simulink model "adcs_sim_finch"  (R2025b)
settings: Solver=VariableStepAuto  StartTime=0.0  StopTime=10.0  RelTol=1e-3
PreLoadFcn:
  | run("sim_config.m")
undefined symbols (not defined in the file or in its folder): MU_EARTH_KM3PS2, sc
libraries: simulink x11
settings Model: Creator=alex  LastModifiedBy=alex

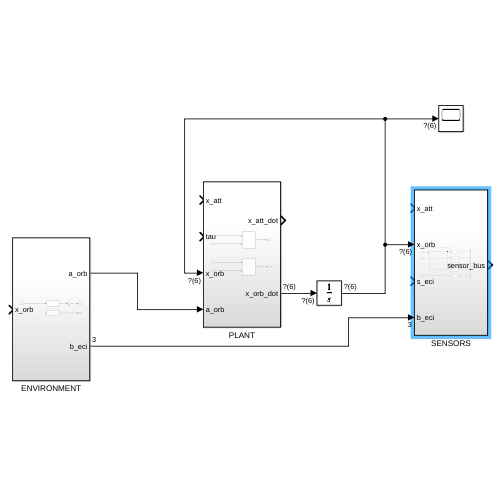
[thumbnail: Simulink's stored preview of the top-level diagram]
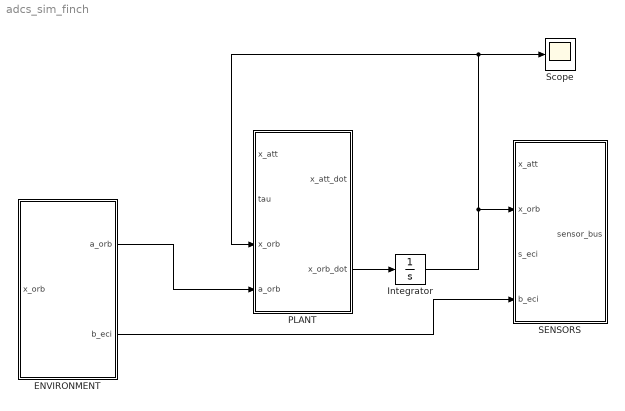
== system adcs_sim_finch ==
  ENVIRONMENT : Subsystem
  Integrator : Integrator
  PLANT : Subsystem
  SENSORS : Subsystem
  Scope : Scope
  wires:
  ENVIRONMENT/1(a_orb) -> PLANT/4(a_orb)
  PLANT/2(x_orb_dot) -> Integrator/1
  Integrator/1 -> SENSORS/2(x_orb), Scope/1, PLANT/3(x_orb)
  ENVIRONMENT/2(b_eci) -> SENSORS/4(b_eci)

== system adcs_sim_finch/ENVIRONMENT ==
  x_orb : Inport
  GEOMAGNETISM : Subsystem
  GRAVITY : Subsystem
  Sum : Sum  Inputs=|++
  a_orb : Outport
  b_eci : Outport  Port=2
  wires:
  x_orb/1 -> GRAVITY/1(x_orb)
  GRAVITY/1(a_grav) -> Sum/1
  Sum/1 -> a_orb/1
  GEOMAGNETISM/1(b) -> b_eci/1

== system adcs_sim_finch/PLANT ==
  x_att : Inport
  tau : Inport  Port=2
  x_orb : Inport  Port=3
  a_orb : Inport  Port=4
  ATTITUDE : Subsystem
  ORBIT : Subsystem
  x_att_dot : Outport
  x_orb_dot : Outport  Port=2
  wires:
  x_att/1 -> ATTITUDE/1(x)
  tau/1 -> ATTITUDE/2(tau)
  x_orb/1 -> ORBIT/1(x_orb)
  ATTITUDE/1(x_dot) -> x_att_dot/1
  ORBIT/1(x_orb_dot) -> x_orb_dot/1
  a_orb/1 -> ORBIT/2(a_orb)

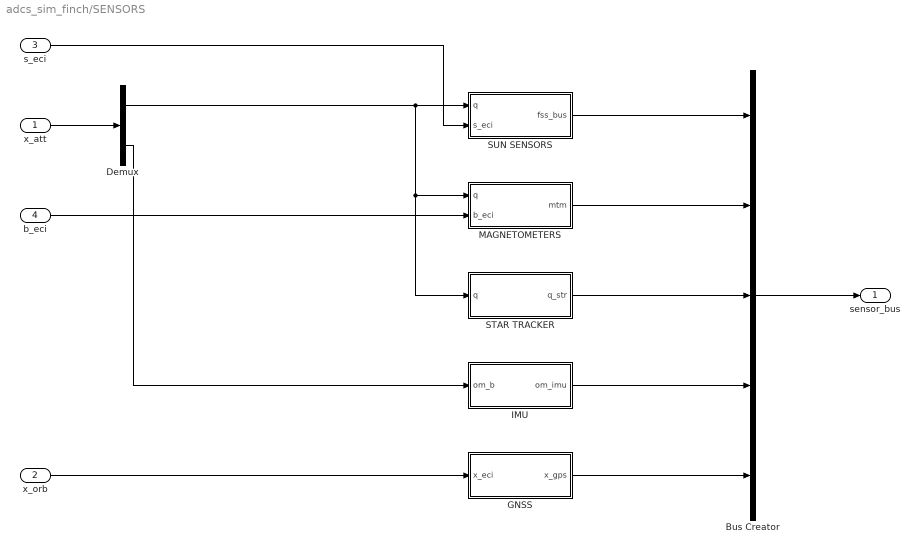
== system adcs_sim_finch/SENSORS ==
  x_att : Inport
  x_orb : Inport  Port=2
  s_eci : Inport  Port=3
  b_eci : Inport  Port=4
  Bus Creator : BusCreator  Inputs=5
  Demux : Demux  Outputs=[4, 3]
  GNSS : Subsystem
  IMU : Subsystem
  MAGNETOMETERS : Subsystem
  STAR TRACKER : Subsystem
  SUN SENSORS : Subsystem
  sensor_bus : Outport
  wires:
  x_att/1 -> Demux/1
  Demux/1 -> STAR TRACKER/1(q), MAGNETOMETERS/1(q), SUN SENSORS/1(q)
  Demux/2 -> IMU/1(om_b)
  x_orb/1 -> GNSS/1(x_eci)
  s_eci/1 -> SUN SENSORS/2(s_eci)
  b_eci/1 -> MAGNETOMETERS/2(b_eci)
  SUN SENSORS/1(fss_bus) -> Bus Creator/1
  GNSS/1(x_gps) -> Bus Creator/5
  IMU/1(om_imu) -> Bus Creator/4
  STAR TRACKER/1(q_str) -> Bus Creator/3
  MAGNETOMETERS/1(mtm) -> Bus Creator/2
  Bus Creator/1 -> sensor_bus/1

== system adcs_sim_finch/ENVIRONMENT/GEOMAGNETISM ==
  x_orb : Inport
  PLACEHOLDER : Constant  Value=[60; 0; 0]
  b : Outport
  wires:
  PLACEHOLDER/1 -> b/1

== system adcs_sim_finch/ENVIRONMENT/GRAVITY ==
  x_orb : Inport
  J2 : Subsystem
  Mux : Mux  Inputs=2
  a_grav : Outport
  wires:
  x_orb/1 -> J2/1(x_orb)
  J2/1(p) -> Mux/1
  Mux/1 -> a_grav/1

== system adcs_sim_finch/PLANT/ATTITUDE ==
  x : Inport
  tau : Inport  Port=2
  DYNAMICS : Subsystem
  Demux : Demux  Outputs=2
  KINEMATICS : Subsystem
  Mux : Mux  Inputs=2
  x_dot : Outport
  wires:
  x/1 -> Demux/1
  Demux/1 -> KINEMATICS/1(q)  "q"
  Demux/2 -> KINEMATICS/2(om_b), DYNAMICS/1(om_b)  "om_b"
  tau/1 -> DYNAMICS/2(tau)
  KINEMATICS/1(q_dot) -> Mux/1
  DYNAMICS/1(om_b_dot) -> Mux/2
  Mux/1 -> x_dot/1

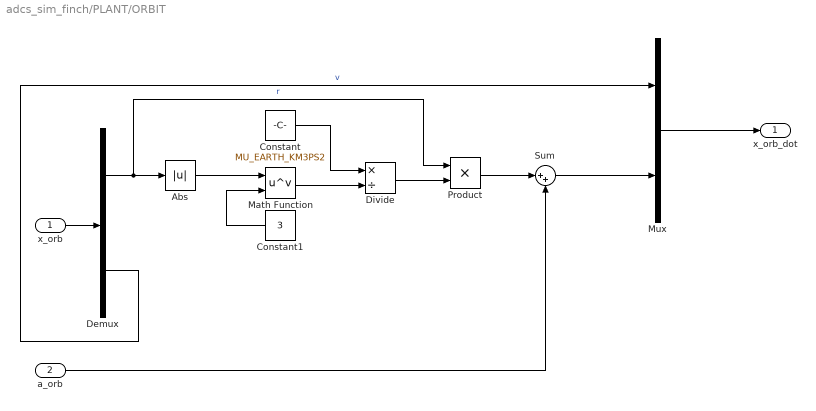
== system adcs_sim_finch/PLANT/ORBIT ==
  x_orb : Inport
  a_orb : Inport  Port=2
  Abs : Abs  SaturateOnIntegerOverflow=off
  Constant : Constant  Value=MU_EARTH_KM3PS2
  Constant1 : Constant  Value=3
  Demux : Demux  Outputs=[3, 3]
  Divide : Product  Inputs=*/
  Math Function : Math  Operator=pow
  Mux : Mux  Inputs=2
  Product : Product
  Sum : Sum  Inputs=|++
  x_orb_dot : Outport
  wires:
  x_orb/1 -> Demux/1
  Mux/1 -> x_orb_dot/1
  Constant1/1 -> Math Function/2
  Demux/1 -> Product/1, Abs/1  "r"
  Abs/1 -> Math Function/1
  Math Function/1 -> Divide/2
  Constant/1 -> Divide/1
  Divide/1 -> Product/2
  Product/1 -> Sum/1
  a_orb/1 -> Sum/2
  Sum/1 -> Mux/2
  Demux/2 -> Mux/1  "v"

== system adcs_sim_finch/SENSORS/GNSS ==
  x_eci : Inport
  Band-Limited White Noise : simulink/Sources/Band-Limited White Noise  Cov=sc.gps.obj.cov ./ (1 / sc.gps.obj.rate)  Ts=1 / sc.gps.obj.rate  seed=[23341]
  Sum : Sum  Inputs=|++
  x_gps : Outport
  wires:
  x_eci/1 -> Sum/1
  Sum/1 -> x_gps/1

== system adcs_sim_finch/SENSORS/IMU ==
  om_b : Inport
  Band-Limited White Noise : simulink/Sources/Band-Limited White Noise  Cov=sc.imu.obj.bias_instability.^2 ./ (1 ./ sc.imu.obj.rate)  Ts=1 / sc.imu.obj.rate  seed=[23341]
  Band-Limited White Noise1 : simulink/Sources/Band-Limited White Noise  Cov=sc.imu.obj.arw.^2  Ts=1 / sc.imu.obj.rate  seed=[23341]
  Integrator : Integrator
  Product : Product  Multiplication=Matrix(*)
  Sum : Sum  Inputs=+++
  sc.imu.dcm : Constant  Value=sc.imu.dcm
  om_imu : Outport
  wires:
  om_b/1 -> Product/2
  sc.imu.dcm/1 -> Product/1
  Product/1 -> Sum/2
  Integrator/1 -> Sum/3  "bias"
  Sum/1 -> om_imu/1

== system adcs_sim_finch/SENSORS/MAGNETOMETERS ==
  q : Inport
  b_eci : Inport  Port=2
  MTM1 : Subsystem
  mtm : Outport
  wires:
  q/1 -> MTM1/1(q)
  b_eci/1 -> MTM1/2(b_eci)
  MTM1/1(b_s) -> mtm/1

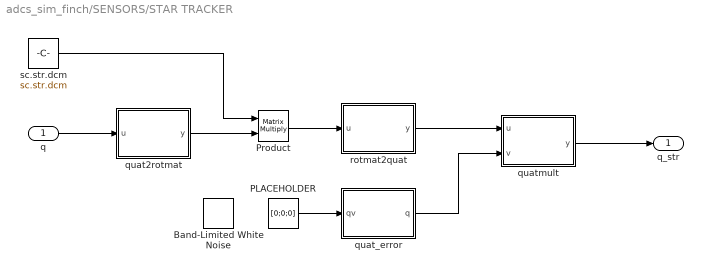
== system adcs_sim_finch/SENSORS/STAR TRACKER ==
  q : Inport
  Band-Limited White Noise : simulink/Sources/Band-Limited White Noise  Cov=sc.str.obj.cov  Ts=1 / sc.str.obj.rate  seed=[23341]
  PLACEHOLDER : Constant  Value=[0;0;0]
  Product : Product  Multiplication=Matrix(*)
  quat2rotmat : MATLAB Function  TreatAsAtomicUnit=on
  quat_error : MATLAB Function  TreatAsAtomicUnit=on
  quatmult : MATLAB Function  TreatAsAtomicUnit=on
  rotmat2quat : MATLAB Function  TreatAsAtomicUnit=on
  sc.str.dcm : Constant  Value=sc.str.dcm
  q_str : Outport
  wires:
  q/1 -> quat2rotmat/1(u)
  quat2rotmat/1(y) -> Product/2
  sc.str.dcm/1 -> Product/1
  Product/1 -> rotmat2quat/1(u)
  rotmat2quat/1(y) -> quatmult/1(u)
  quat_error/1(q) -> quatmult/2(v)
  quatmult/1(y) -> q_str/1
  PLACEHOLDER/1 -> quat_error/1(qv)

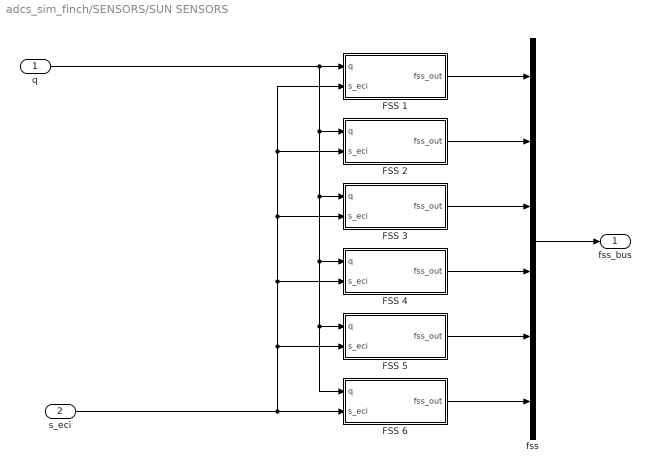
== system adcs_sim_finch/SENSORS/SUN SENSORS ==
  q : Inport
  s_eci : Inport  Port=2
  FSS 1 : Subsystem
  FSS 2 : Subsystem
  FSS 3 : Subsystem
  FSS 4 : Subsystem
  FSS 5 : Subsystem
  FSS 6 : Subsystem
  fss : BusCreator  Inputs=6
  fss_bus : Outport
  wires:
  FSS 1/1(fss_out) -> fss/1
  FSS 2/1(fss_out) -> fss/2
  FSS 3/1(fss_out) -> fss/3
  FSS 4/1(fss_out) -> fss/4
  FSS 5/1(fss_out) -> fss/5
  FSS 6/1(fss_out) -> fss/6
  q/1 -> FSS 5/1(q), FSS 6/1(q), FSS 4/1(q), FSS 3/1(q), FSS 2/1(q), FSS 1/1(q)
  s_eci/1 -> FSS 1/2(s_eci), FSS 2/2(s_eci), FSS 3/2(s_eci), FSS 4/2(s_eci), FSS 5/2(s_eci), FSS 6/2(s_eci)
  fss/1 -> fss_bus/1

== system adcs_sim_finch/ENVIRONMENT/GRAVITY/J2 ==
  x_orb : Inport
  J2 acceleration : MATLAB Function  TreatAsAtomicUnit=on
  p : Outport
  wires:
  x_orb/1 -> J2 acceleration/1(x)
  J2 acceleration/1(p) -> p/1

== system adcs_sim_finch/PLANT/ATTITUDE/DYNAMICS ==
  om_b : Inport
  tau : Inport  Port=2
  Constant : Constant  Value=sc.moi
  Product : Product  Inputs=3  Multiplication=Matrix(*)
  Product1 : Product  Multiplication=Matrix(*)
  Sum : Sum  Inputs=-+|
  sc.moi_inv : Constant  Value=sc.moi_inv
  skew3 : MATLAB Function  TreatAsAtomicUnit=on
  om_b_dot : Outport
  wires:
  om_b/1 -> Product/2, skew3/1(u)
  skew3/1(y) -> Product/3
  Constant/1 -> Product/1
  tau/1 -> Sum/2
  Product/1 -> Sum/1
  Sum/1 -> Product1/2
  sc.moi_inv/1 -> Product1/1
  Product1/1 -> om_b_dot/1

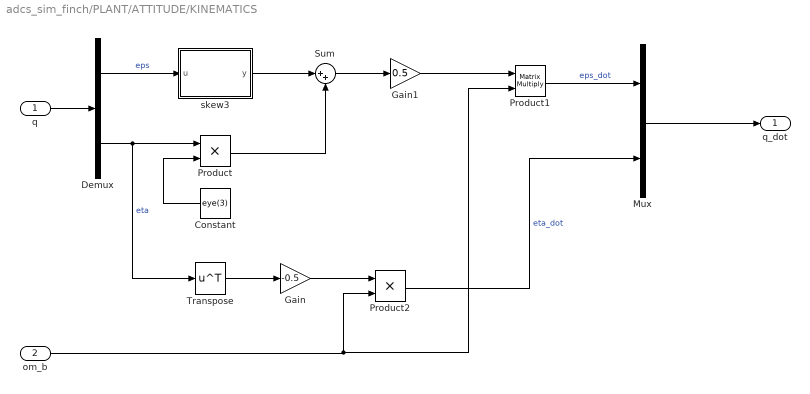
== system adcs_sim_finch/PLANT/ATTITUDE/KINEMATICS ==
  q : Inport
  om_b : Inport  Port=2
  Constant : Constant  Value=eye(3)
  Demux : Demux  Outputs=[3, 1]
  Gain : Gain  Gain=-0.5
  Gain1 : Gain  Gain=0.5
  Mux : Mux  Inputs=2
  Product : Product
  Product1 : Product  Multiplication=Matrix(*)
  Product2 : Product
  Sum : Sum  Inputs=|++
  Transpose : Math  Operator=transpose
  skew3 : MATLAB Function  TreatAsAtomicUnit=on
  q_dot : Outport
  wires:
  q/1 -> Demux/1
  Transpose/1 -> Gain/1
  Demux/1 -> skew3/1(u)  "eps"
  skew3/1(y) -> Sum/1
  Demux/2 -> Transpose/1, Product/1  "eta"
  Constant/1 -> Product/2
  Product/1 -> Sum/2
  Sum/1 -> Gain1/1
  Gain1/1 -> Product1/1
  Product1/1 -> Mux/1  "eps_dot"
  Gain/1 -> Product2/1
  om_b/1 -> Product1/2, Product2/2
  Product2/1 -> Mux/2  "eta_dot"
  Mux/1 -> q_dot/1

== system adcs_sim_finch/SENSORS/MAGNETOMETERS/MTM1 ==
  q : Inport
  b_eci : Inport  Port=2
  Band-Limited White Noise : simulink/Sources/Band-Limited White Noise  Cov=sc.mtm1.obj.cov ./ (1 / sc.mtm1.obj.rate)  Ts=1 / sc.mtm1.obj.rate  seed=[23341]
  Product : Product  Multiplication=Matrix(*)
  Product1 : Product  Multiplication=Matrix(*)
  Saturation : Saturate  UpperLimit=sc.mtm1.obj.range(2)  LowerLimit=sc.mtm1.obj.range(1)
  Sum : Sum  Inputs=|++
  quat2rotmat : MATLAB Function  TreatAsAtomicUnit=on
  sc.mtm1.dcm : Constant  Value=sc.mtm1.dcm
  b_s : Outport
  wires:
  q/1 -> quat2rotmat/1(u)
  Product/1 -> Product1/2
  sc.mtm1.dcm/1 -> Product1/1
  Product1/1 -> Sum/1
  Sum/1 -> Saturation/1
  Saturation/1 -> b_s/1
  b_eci/1 -> Product/2
  quat2rotmat/1(y) -> Product/1

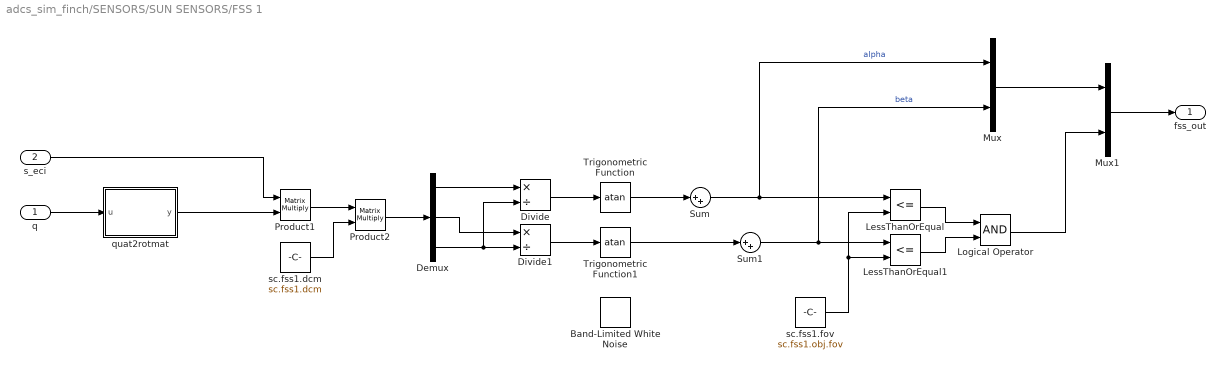
== system adcs_sim_finch/SENSORS/SUN SENSORS/FSS 1 ==
  q : Inport
  s_eci : Inport  Port=2
  Band-Limited White Noise : simulink/Sources/Band-Limited White Noise  Cov=sc.fss1.obj.cov ./ (1 / sc.fss1.obj.rate)  Ts=1 / sc.fss1.obj.rate  seed=[23341]
  Demux : Demux  Outputs=3
  Divide : Product  Inputs=*/
  Divide1 : Product  Inputs=*/
  LessThanOrEqual : RelationalOperator  Operator=<=  OutDataTypeStr=boolean  RndMeth=Simplest  InputSameDT=off
  LessThanOrEqual1 : RelationalOperator  Operator=<=  OutDataTypeStr=boolean  RndMeth=Simplest  InputSameDT=off
  Logical Operator : Logic  AllPortsSameDT=off  OutDataTypeStr=boolean
  Mux : Mux  Inputs=2
  Mux1 : Mux  Inputs=2
  Product1 : Product  Multiplication=Matrix(*)
  Product2 : Product  Multiplication=Matrix(*)
  Sum : Sum  Inputs=|++
  Sum1 : Sum  Inputs=|++
  Trigonometric Function : Trigonometry  Operator=atan
  Trigonometric Function1 : Trigonometry  Operator=atan
  quat2rotmat : MATLAB Function  TreatAsAtomicUnit=on
  sc.fss1.dcm : Constant  Value=sc.fss1.dcm
  sc.fss1.fov : Constant  Value=sc.fss1.obj.fov
  fss_out : Outport
  wires:
  q/1 -> quat2rotmat/1(u)
  quat2rotmat/1(y) -> Product1/2
  sc.fss1.dcm/1 -> Product2/2
  s_eci/1 -> Product1/1
  Product1/1 -> Product2/1
  Product2/1 -> Demux/1
  Demux/1 -> Divide/1
  Demux/3 -> Divide1/2, Divide/2
  Divide/1 -> Trigonometric Function/1
  Demux/2 -> Divide1/1
  Divide1/1 -> Trigonometric Function1/1
  Trigonometric Function/1 -> Sum/1
  Trigonometric Function1/1 -> Sum1/1
  Sum/1 -> Mux/1, LessThanOrEqual/1  "alpha"
  sc.fss1.fov/1 -> LessThanOrEqual1/2, LessThanOrEqual/2
  Sum1/1 -> Mux/2, LessThanOrEqual1/1  "beta"
  LessThanOrEqual/1 -> Logical Operator/1
  LessThanOrEqual1/1 -> Logical Operator/2
  Mux/1 -> Mux1/1
  Logical Operator/1 -> Mux1/2
  Mux1/1 -> fss_out/1

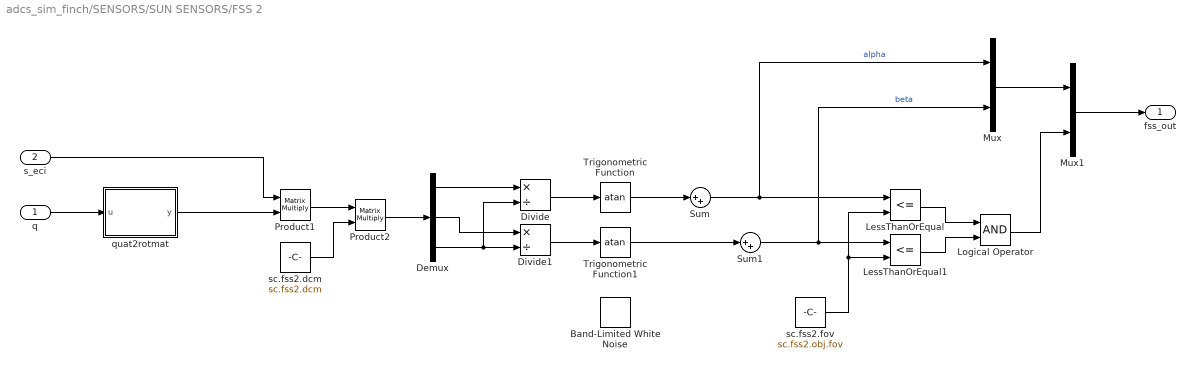
== system adcs_sim_finch/SENSORS/SUN SENSORS/FSS 2 ==
  q : Inport
  s_eci : Inport  Port=2
  Band-Limited White Noise : simulink/Sources/Band-Limited White Noise  Cov=sc.fss2.obj.cov ./ (1 / sc.fss2.obj.rate)  Ts=1 / sc.fss2.obj.rate  seed=[23341]
  Demux : Demux  Outputs=3
  Divide : Product  Inputs=*/
  Divide1 : Product  Inputs=*/
  LessThanOrEqual : RelationalOperator  Operator=<=  OutDataTypeStr=boolean  RndMeth=Simplest  InputSameDT=off
  LessThanOrEqual1 : RelationalOperator  Operator=<=  OutDataTypeStr=boolean  RndMeth=Simplest  InputSameDT=off
  Logical Operator : Logic  AllPortsSameDT=off  OutDataTypeStr=boolean
  Mux : Mux  Inputs=2
  Mux1 : Mux  Inputs=2
  Product1 : Product  Multiplication=Matrix(*)
  Product2 : Product  Multiplication=Matrix(*)
  Sum : Sum  Inputs=|++
  Sum1 : Sum  Inputs=|++
  Trigonometric Function : Trigonometry  Operator=atan
  Trigonometric Function1 : Trigonometry  Operator=atan
  quat2rotmat : MATLAB Function  TreatAsAtomicUnit=on
  sc.fss2.dcm : Constant  Value=sc.fss2.dcm
  sc.fss2.fov : Constant  Value=sc.fss2.obj.fov
  fss_out : Outport
  wires:
  q/1 -> quat2rotmat/1(u)
  quat2rotmat/1(y) -> Product1/2
  sc.fss2.dcm/1 -> Product2/2
  s_eci/1 -> Product1/1
  Product1/1 -> Product2/1
  Product2/1 -> Demux/1
  Demux/1 -> Divide/1
  Demux/3 -> Divide1/2, Divide/2
  Divide/1 -> Trigonometric Function/1
  Demux/2 -> Divide1/1
  Divide1/1 -> Trigonometric Function1/1
  Trigonometric Function/1 -> Sum/1
  Trigonometric Function1/1 -> Sum1/1
  Sum/1 -> Mux/1, LessThanOrEqual/1  "alpha"
  sc.fss2.fov/1 -> LessThanOrEqual1/2, LessThanOrEqual/2
  Sum1/1 -> Mux/2, LessThanOrEqual1/1  "beta"
  LessThanOrEqual/1 -> Logical Operator/1
  LessThanOrEqual1/1 -> Logical Operator/2
  Mux/1 -> Mux1/1
  Logical Operator/1 -> Mux1/2
  Mux1/1 -> fss_out/1

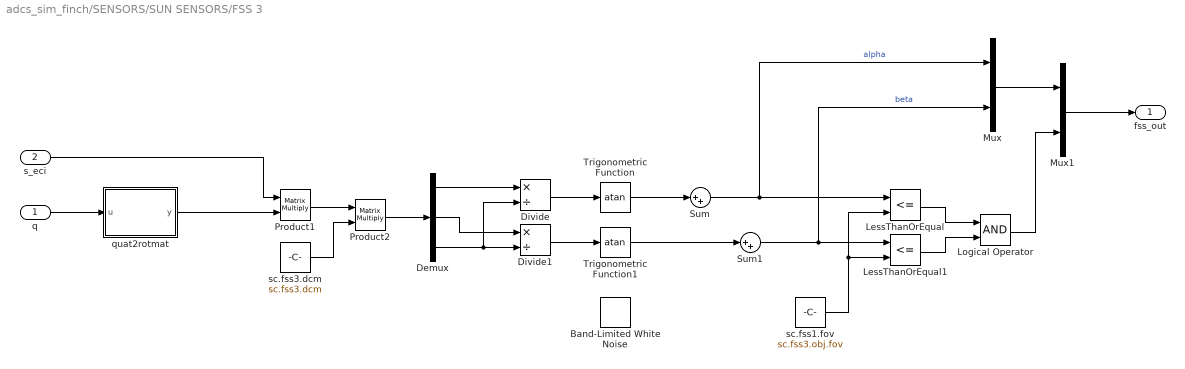
== system adcs_sim_finch/SENSORS/SUN SENSORS/FSS 3 ==
  q : Inport
  s_eci : Inport  Port=2
  Band-Limited White Noise : simulink/Sources/Band-Limited White Noise  Cov=sc.fss3.obj.cov ./ (1 / sc.fss3.obj.rate)  Ts=1 / sc.fss3.obj.rate  seed=[23341]
  Demux : Demux  Outputs=3
  Divide : Product  Inputs=*/
  Divide1 : Product  Inputs=*/
  LessThanOrEqual : RelationalOperator  Operator=<=  OutDataTypeStr=boolean  RndMeth=Simplest  InputSameDT=off
  LessThanOrEqual1 : RelationalOperator  Operator=<=  OutDataTypeStr=boolean  RndMeth=Simplest  InputSameDT=off
  Logical Operator : Logic  AllPortsSameDT=off  OutDataTypeStr=boolean
  Mux : Mux  Inputs=2
  Mux1 : Mux  Inputs=2
  Product1 : Product  Multiplication=Matrix(*)
  Product2 : Product  Multiplication=Matrix(*)
  Sum : Sum  Inputs=|++
  Sum1 : Sum  Inputs=|++
  Trigonometric Function : Trigonometry  Operator=atan
  Trigonometric Function1 : Trigonometry  Operator=atan
  quat2rotmat : MATLAB Function  TreatAsAtomicUnit=on
  sc.fss1.fov : Constant  Value=sc.fss3.obj.fov
  sc.fss3.dcm : Constant  Value=sc.fss3.dcm
  fss_out : Outport
  wires:
  q/1 -> quat2rotmat/1(u)
  quat2rotmat/1(y) -> Product1/2
  sc.fss3.dcm/1 -> Product2/2
  s_eci/1 -> Product1/1
  Product1/1 -> Product2/1
  Product2/1 -> Demux/1
  Demux/1 -> Divide/1
  Demux/3 -> Divide1/2, Divide/2
  Divide/1 -> Trigonometric Function/1
  Demux/2 -> Divide1/1
  Divide1/1 -> Trigonometric Function1/1
  Trigonometric Function/1 -> Sum/1
  Trigonometric Function1/1 -> Sum1/1
  Sum/1 -> Mux/1, LessThanOrEqual/1  "alpha"
  sc.fss1.fov/1 -> LessThanOrEqual1/2, LessThanOrEqual/2
  Sum1/1 -> Mux/2, LessThanOrEqual1/1  "beta"
  LessThanOrEqual/1 -> Logical Operator/1
  LessThanOrEqual1/1 -> Logical Operator/2
  Mux/1 -> Mux1/1
  Logical Operator/1 -> Mux1/2
  Mux1/1 -> fss_out/1

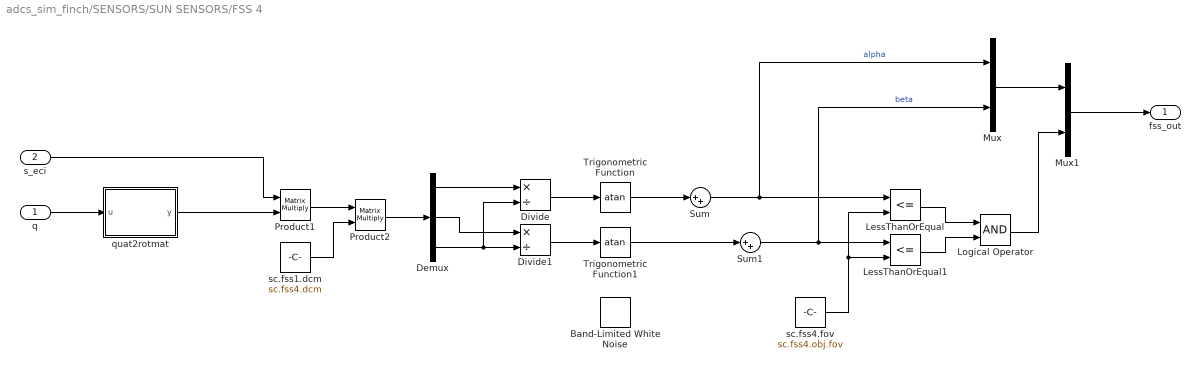
== system adcs_sim_finch/SENSORS/SUN SENSORS/FSS 4 ==
  q : Inport
  s_eci : Inport  Port=2
  Band-Limited White Noise : simulink/Sources/Band-Limited White Noise  Cov=sc.fss4.obj.cov ./ (1 / sc.fss4.obj.rate)  Ts=1 / sc.fss4.obj.rate  seed=[23341]
  Demux : Demux  Outputs=3
  Divide : Product  Inputs=*/
  Divide1 : Product  Inputs=*/
  LessThanOrEqual : RelationalOperator  Operator=<=  OutDataTypeStr=boolean  RndMeth=Simplest  InputSameDT=off
  LessThanOrEqual1 : RelationalOperator  Operator=<=  OutDataTypeStr=boolean  RndMeth=Simplest  InputSameDT=off
  Logical Operator : Logic  AllPortsSameDT=off  OutDataTypeStr=boolean
  Mux : Mux  Inputs=2
  Mux1 : Mux  Inputs=2
  Product1 : Product  Multiplication=Matrix(*)
  Product2 : Product  Multiplication=Matrix(*)
  Sum : Sum  Inputs=|++
  Sum1 : Sum  Inputs=|++
  Trigonometric Function : Trigonometry  Operator=atan
  Trigonometric Function1 : Trigonometry  Operator=atan
  quat2rotmat : MATLAB Function  TreatAsAtomicUnit=on
  sc.fss1.dcm : Constant  Value=sc.fss4.dcm
  sc.fss4.fov : Constant  Value=sc.fss4.obj.fov
  fss_out : Outport
  wires:
  q/1 -> quat2rotmat/1(u)
  quat2rotmat/1(y) -> Product1/2
  sc.fss1.dcm/1 -> Product2/2
  s_eci/1 -> Product1/1
  Product1/1 -> Product2/1
  Product2/1 -> Demux/1
  Demux/1 -> Divide/1
  Demux/3 -> Divide1/2, Divide/2
  Divide/1 -> Trigonometric Function/1
  Demux/2 -> Divide1/1
  Divide1/1 -> Trigonometric Function1/1
  Trigonometric Function/1 -> Sum/1
  Trigonometric Function1/1 -> Sum1/1
  Sum/1 -> Mux/1, LessThanOrEqual/1  "alpha"
  sc.fss4.fov/1 -> LessThanOrEqual1/2, LessThanOrEqual/2
  Sum1/1 -> Mux/2, LessThanOrEqual1/1  "beta"
  LessThanOrEqual/1 -> Logical Operator/1
  LessThanOrEqual1/1 -> Logical Operator/2
  Mux/1 -> Mux1/1
  Logical Operator/1 -> Mux1/2
  Mux1/1 -> fss_out/1

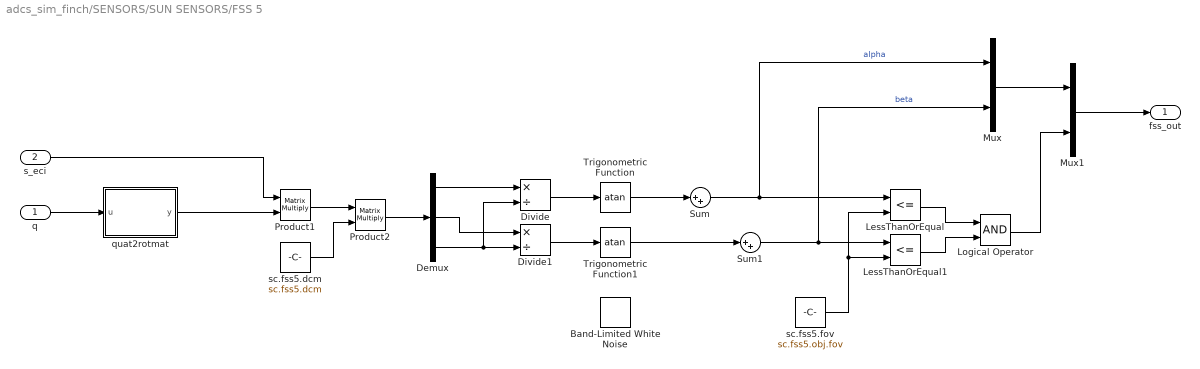
== system adcs_sim_finch/SENSORS/SUN SENSORS/FSS 5 ==
  q : Inport
  s_eci : Inport  Port=2
  Band-Limited White Noise : simulink/Sources/Band-Limited White Noise  Cov=sc.fss5.obj.cov ./ (1 / sc.fss5.obj.rate)  Ts=1 / sc.fss5.obj.rate  seed=[23341]
  Demux : Demux  Outputs=3
  Divide : Product  Inputs=*/
  Divide1 : Product  Inputs=*/
  LessThanOrEqual : RelationalOperator  Operator=<=  OutDataTypeStr=boolean  RndMeth=Simplest  InputSameDT=off
  LessThanOrEqual1 : RelationalOperator  Operator=<=  OutDataTypeStr=boolean  RndMeth=Simplest  InputSameDT=off
  Logical Operator : Logic  AllPortsSameDT=off  OutDataTypeStr=boolean
  Mux : Mux  Inputs=2
  Mux1 : Mux  Inputs=2
  Product1 : Product  Multiplication=Matrix(*)
  Product2 : Product  Multiplication=Matrix(*)
  Sum : Sum  Inputs=|++
  Sum1 : Sum  Inputs=|++
  Trigonometric Function : Trigonometry  Operator=atan
  Trigonometric Function1 : Trigonometry  Operator=atan
  quat2rotmat : MATLAB Function  TreatAsAtomicUnit=on
  sc.fss5.dcm : Constant  Value=sc.fss5.dcm
  sc.fss5.fov : Constant  Value=sc.fss5.obj.fov
  fss_out : Outport
  wires:
  q/1 -> quat2rotmat/1(u)
  quat2rotmat/1(y) -> Product1/2
  sc.fss5.dcm/1 -> Product2/2
  s_eci/1 -> Product1/1
  Product1/1 -> Product2/1
  Product2/1 -> Demux/1
  Demux/1 -> Divide/1
  Demux/3 -> Divide1/2, Divide/2
  Divide/1 -> Trigonometric Function/1
  Demux/2 -> Divide1/1
  Divide1/1 -> Trigonometric Function1/1
  Trigonometric Function/1 -> Sum/1
  Trigonometric Function1/1 -> Sum1/1
  Sum/1 -> Mux/1, LessThanOrEqual/1  "alpha"
  sc.fss5.fov/1 -> LessThanOrEqual1/2, LessThanOrEqual/2
  Sum1/1 -> Mux/2, LessThanOrEqual1/1  "beta"
  LessThanOrEqual/1 -> Logical Operator/1
  LessThanOrEqual1/1 -> Logical Operator/2
  Mux/1 -> Mux1/1
  Logical Operator/1 -> Mux1/2
  Mux1/1 -> fss_out/1

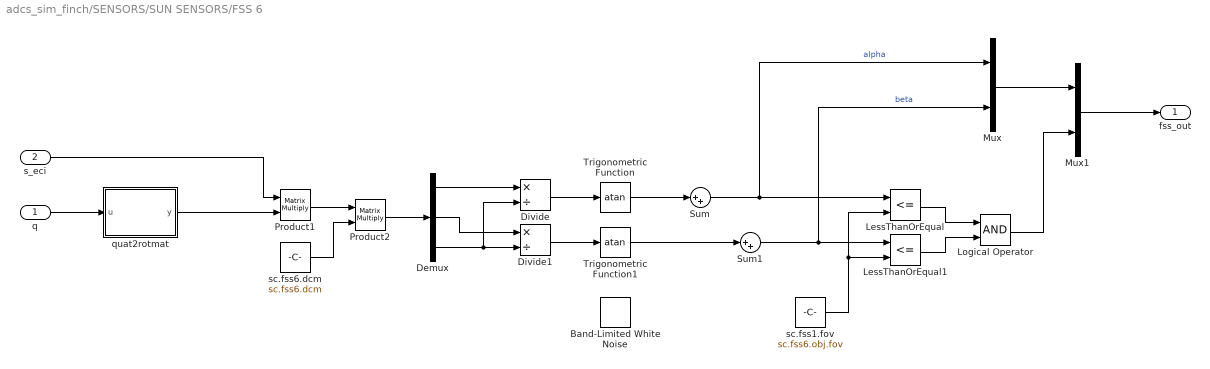
== system adcs_sim_finch/SENSORS/SUN SENSORS/FSS 6 ==
  q : Inport
  s_eci : Inport  Port=2
  Band-Limited White Noise : simulink/Sources/Band-Limited White Noise  Cov=sc.fss6.obj.cov ./ (1 / sc.fss6.obj.rate)  Ts=1 / sc.fss6.obj.rate  seed=[23341]
  Demux : Demux  Outputs=3
  Divide : Product  Inputs=*/
  Divide1 : Product  Inputs=*/
  LessThanOrEqual : RelationalOperator  Operator=<=  OutDataTypeStr=boolean  RndMeth=Simplest  InputSameDT=off
  LessThanOrEqual1 : RelationalOperator  Operator=<=  OutDataTypeStr=boolean  RndMeth=Simplest  InputSameDT=off
  Logical Operator : Logic  AllPortsSameDT=off  OutDataTypeStr=boolean
  Mux : Mux  Inputs=2
  Mux1 : Mux  Inputs=2
  Product1 : Product  Multiplication=Matrix(*)
  Product2 : Product  Multiplication=Matrix(*)
  Sum : Sum  Inputs=|++
  Sum1 : Sum  Inputs=|++
  Trigonometric Function : Trigonometry  Operator=atan
  Trigonometric Function1 : Trigonometry  Operator=atan
  quat2rotmat : MATLAB Function  TreatAsAtomicUnit=on
  sc.fss1.fov : Constant  Value=sc.fss6.obj.fov
  sc.fss6.dcm : Constant  Value=sc.fss6.dcm
  fss_out : Outport
  wires:
  q/1 -> quat2rotmat/1(u)
  quat2rotmat/1(y) -> Product1/2
  sc.fss6.dcm/1 -> Product2/2
  s_eci/1 -> Product1/1
  Product1/1 -> Product2/1
  Product2/1 -> Demux/1
  Demux/1 -> Divide/1
  Demux/3 -> Divide1/2, Divide/2
  Divide/1 -> Trigonometric Function/1
  Demux/2 -> Divide1/1
  Divide1/1 -> Trigonometric Function1/1
  Trigonometric Function/1 -> Sum/1
  Trigonometric Function1/1 -> Sum1/1
  Sum/1 -> Mux/1, LessThanOrEqual/1  "alpha"
  sc.fss1.fov/1 -> LessThanOrEqual1/2, LessThanOrEqual/2
  Sum1/1 -> Mux/2, LessThanOrEqual1/1  "beta"
  LessThanOrEqual/1 -> Logical Operator/1
  LessThanOrEqual1/1 -> Logical Operator/2
  Mux/1 -> Mux1/1
  Logical Operator/1 -> Mux1/2
  Mux1/1 -> fss_out/1

== matlab function adcs_sim_finch/ENVIRONMENT/GRAVITY/J2/J2 acceleration ==
  data: x input; p output
function p = fcn(x)

% Position vector norm
r = norm(x);

% Common premultiplier
k = (3 / 2) * (J2_EARTH * MU_EARTH_KM3PS2 * EQ_RAD^2) / r^4;

% Perturbation in x
px = k * (x(1) / r) * (5 * (x(3)^2 / r^2) - 1);
% Perturbation in y
py = k * (x(2) / r) * (5 * (x(3)^2 / r^2) - 1);
% Perturbation in z
pz = k * (x(3) / r) * (5 * (x(3)^2 / r^2) - 3);

p = [px; py; pz];

== matlab function adcs_sim_finch/PLANT/ATTITUDE/KINEMATICS/skew3 ==
  data: u input; y output
function y = fcn(u)
y = skew3(u);
y = u;

== matlab function adcs_sim_finch/SENSORS/SUN SENSORS/FSS 1/quat2rotmat ==
  data: u input; y output
function y = fcn(u)
y = quat2rotmat(u);

== matlab function adcs_sim_finch/SENSORS/SUN SENSORS/FSS 2/quat2rotmat ==
  data: u input; y output
function y = fcn(u)
y = quat2rotmat(u);

== matlab function adcs_sim_finch/SENSORS/SUN SENSORS/FSS 3/quat2rotmat ==
  data: u input; y output
function y = fcn(u)
y = quat2rotmat(u);

== matlab function adcs_sim_finch/SENSORS/SUN SENSORS/FSS 4/quat2rotmat ==
  data: u input; y output
function y = fcn(u)
y = quat2rotmat(u);

== matlab function adcs_sim_finch/SENSORS/SUN SENSORS/FSS 5/quat2rotmat ==
  data: u input; y output
function y = fcn(u)
y = quat2rotmat(u);

== matlab function adcs_sim_finch/SENSORS/SUN SENSORS/FSS 6/quat2rotmat ==
  data: u input; y output
function y = fcn(u)
y = quat2rotmat(u);

== matlab function adcs_sim_finch/SENSORS/MAGNETOMETERS/MTM1/quat2rotmat ==
  data: u input; y output
function y = fcn(u)
y = quat2rotmat(u);

== matlab function adcs_sim_finch/SENSORS/STAR TRACKER/quat2rotmat ==
  data: u input; y output
function y = fcn(u)
y = quat2rotmat(u);

== matlab function adcs_sim_finch/SENSORS/STAR TRACKER/rotmat2quat ==
  data: u input; y output
function y = fcn(u)
y = rotmat2quat(u);

== matlab function adcs_sim_finch/PLANT/ATTITUDE/DYNAMICS/skew3 ==
  data: u input; y output
function y = fcn(u)
y = skew3(u);
y = u;

== matlab function adcs_sim_finch/SENSORS/STAR TRACKER/quatmult ==
  data: u input; y output; v input
function y = fcn(u, v)
y = quatmult(u, v);

== matlab function adcs_sim_finch/SENSORS/STAR TRACKER/quat_error ==
  data: qv input; q output
function q = fcn(qv)
% Compute the error quaternion scalar component and return full error
% quaternion
qw = sqrt(1 - 0.25 * norm(qv)^2);
q = [0.5 .* qv; qw];
